simulink model "pendulum_on_a_cart_ctrl"  (R2020a)
settings: Solver=daessc  StartTime=0.0  StopTime=simlength  MaxStep=ts  RelTol=1e-3
values from neighbouring files (symbols this model uses):
  A = [0 1 0 0;      0 -b0*(J1+m1*s1^2)/den  -g*m1^2*s1^2/den b1*m1*s1/den;      0 0 0 1;      0 b0*m1*s1/den g*m1*(m0+m1)*s1/den -b1*(m0+m1)/den]    [init_pendulum_on_a_cart_ctrl.m]
  B = [0 (J1+m1*s1^2)/den 0 -m1*s1/den]'    [init_pendulum_on_a_cart_ctrl.m]
  C = [1 0 0 0; 0 0 1 0]    [init_pendulum_on_a_cart_ctrl.m]
  g = 9.8    [init_pendulum_on_a_cart_ctrl.m]
  Ke = acker(Ae,Be,poles_sf)    [init_pendulum_on_a_cart_ctrl.m]
  L = (place(A',C',poles_obs))'    [init_pendulum_on_a_cart_ctrl.m]
libraries: nesl_utility x6, pendulum_on_a_cart_lib x1
settings Model: Creator=dbagn  LastModifiedBy=dbagn
settings DataIOCC: ReturnWorkspaceOutputs=off

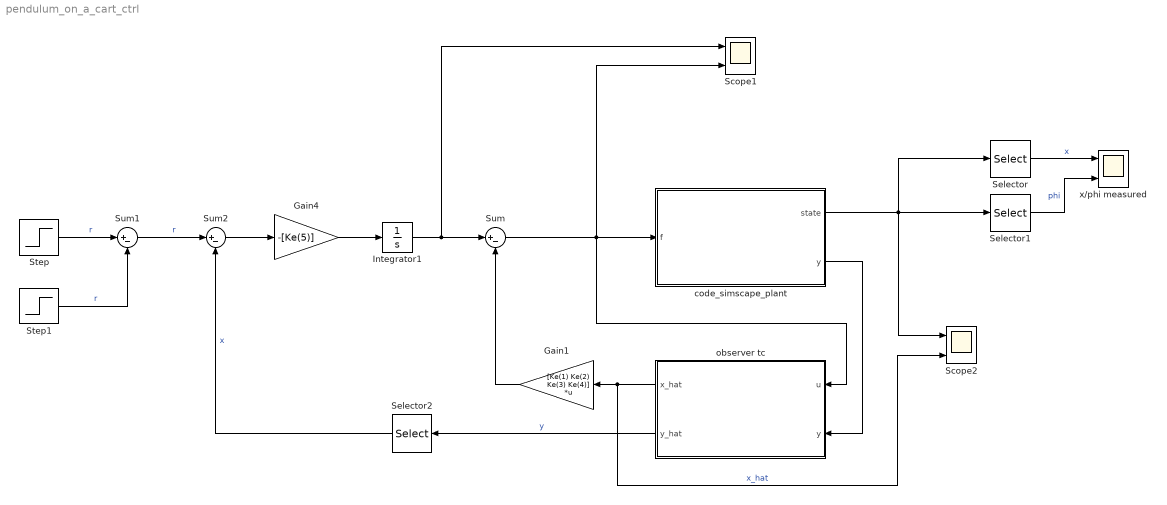
== system pendulum_on_a_cart_ctrl ==
  Gain1 : Gain  Gain=[Ke(1) Ke(2) Ke(3) Ke(4)]  Multiplication=Matrix(K*u)
  Gain4 : Gain  Gain=-[Ke(5)]
  Integrator1 : Integrator
  Scope1 : Scope  NumInputPorts=2
  Scope2 : Scope  NumInputPorts=2
  Selector : Selector  InputPortWidth=4  IndexOptions=Index vector (dialog)  Indices=1  OutputSizes=1
  Selector1 : Selector  InputPortWidth=4  IndexOptions=Index vector (dialog)  Indices=3  OutputSizes=1
  Selector2 : Selector  InputPortWidth=2  IndexOptions=Index vector (dialog)  Indices=1  OutputSizes=1
  Step : Step  SampleTime=0
  Step1 : Step  Time=8  After=2  SampleTime=0
  Sum : Sum  Inputs=|+-
  Sum1 : Sum  Inputs=|+-
  Sum2 : Sum  Inputs=|+-
  "code_simscape_plant " : Subsystem
  observer tc : Subsystem
  x/phi measured : Scope  NumInputPorts=2
  wires:
  Selector/1 -> x/phi measured/1  "x"
  Integrator1/1 -> Sum/1, Scope1/1
  "code_simscape_plant "/2(y) -> observer tc/2(y)
  observer tc/2(y_hat) -> Selector2/1  "y"
  Sum1/1 -> Sum2/1  "r"
  Gain4/1 -> Integrator1/1
  Sum2/1 -> Gain4/1
  Selector1/1 -> x/phi measured/2  "phi"
  Sum/1 -> Scope1/2, observer tc/1(u), "code_simscape_plant "/1(f)
  "code_simscape_plant "/1(state) -> Selector/1, Scope2/1, Selector1/1
  Gain1/1 -> Sum/2
  observer tc/1(x_hat) -> Scope2/2, Gain1/1  "x_hat"
  Selector2/1 -> Sum2/2  "x"
  Step/1 -> Sum1/1  "r"
  Step1/1 -> Sum1/2  "r"

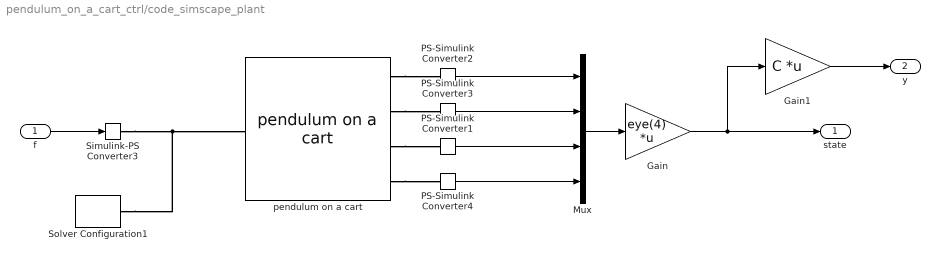
== system pendulum_on_a_cart_ctrl/code_simscape_plant  ==
  f : Inport
  Gain : Gain  Gain=eye(4)  Multiplication=Matrix(K*u)
  Gain1 : Gain  Gain=C  Multiplication=Matrix(K*u)
  Mux : Mux
  PS-Simulink Converter1 : nesl_utility/PS-Simulink Converter  PhysicalDomain=network_engine_domain  SubClassName=ps_output  LeftPortType=input  RightPortType=output  PseudoPeriodic=off  Frequencies=[]  Unit=rad  AffineConversion=on
  PS-Simulink Converter2 : nesl_utility/PS-Simulink Converter  PhysicalDomain=network_engine_domain  SubClassName=ps_output  LeftPortType=input  RightPortType=output  PseudoPeriodic=off  Frequencies=[]  Unit=m  AffineConversion=on
  PS-Simulink Converter3 : nesl_utility/PS-Simulink Converter  PhysicalDomain=network_engine_domain  SubClassName=ps_output  LeftPortType=input  RightPortType=output  PseudoPeriodic=off  Frequencies=[]  Unit=m/s  AffineConversion=on
  PS-Simulink Converter4 : nesl_utility/PS-Simulink Converter  PhysicalDomain=network_engine_domain  SubClassName=ps_output  LeftPortType=input  RightPortType=output  PseudoPeriodic=off  Frequencies=[]  Unit=rad/s  AffineConversion=on
  Simulink-PS Converter3 : nesl_utility/Simulink-PS Converter  PhysicalDomain=network_engine_domain  SubClassName=ps_input  LeftPortType=input  RightPortType=output  PseudoPeriodic=off  Frequencies=[]  NoiseDistribution=none  NoiseParameters=[]  Unit=N  AffineConversion=off  FilteringAndDerivatives=provide  SimscapeFilterOrder=1  InputFilterTimeConstant=0.001  UdotUserProvided=0
  Solver Configuration1 : nesl_utility/Solver Configuration  PhysicalDomain=network_engine_domain  SubClassName=solver  LeftPortType=input  RightPortType=generic  Tones=[]  Harmonics=[]  SimulateNoise=off  Profile=off  UseLocalSampling=off  EnableSwitchedLinearOptims=on  FrequencyDomain=off  UseCCode=off  RelTol=0.001  AbsTol=1e-06  MinStep=1e-09  ToWorkspace=off  RevertToSquareIcSolve=off  NumHomotopyIterations=100  PhasorMode=off  PhasorModeNumHarmonics=1  DoDC=on  ResidualTolerance=1e-09  UseLocalSolver=off  LocalSolverChoice=NE_BACKWARD_EULER_ADVANCER  LocalSolverSampleTime=ts  DoFixedCost=off  MaxNonlinIter=3  MaxModeIter=2  LinearAlgebra=auto  EquationFormulation=NE_TIME_EF  DelaysMemoryBudget=1024  AutomaticFiltering=on  FilteringTimeConstant=0.001  PartitionStorageMethod=AS_NEEDED  PartitionMemoryBudget=1024  PartitionMethod=ROBUST
  pendulum on a cart : pendulum_on_a_cart_lib/pendulum on a cart  m0=m0 kg  m1=m1 kg  J1=J1 kg*m^2  s1=s1 m  b0=b0 N/(m/s)  b1=b1 N*m/(rad/s)  g=g m/s^2  x1_specify=off  x1_priority=High  x1=0 m  x1_nominal_specify=off  x1_nominal_unit=m  x1_nominal_value=1  x2_specify=off  x2_priority=High  x2=0 m/s  x2_nominal_specify=off  x2_nominal_unit=m/s  x2_nominal_value=1  x3_specify=off  x3_priority=High  x3=pi rad  x3_nominal_specify=off  x3_nominal_unit=rad  x3_nominal_value=1  x4_specify=off  x4_priority=High  x4=0 rad/s  x4_nominal_specify=off  x4_nominal_unit=rad/s  x4_nominal_value=1
      settings: InternalSimscapePortConfiguration="{\"Bottom\":[],\"Left\":[{\"id\":\"f\",\"label\":\"f\",\"type\":\"input\"}],\"Right\":[{\"id\":\"x\",\"label\":\"x\",\"type\":\"output\"},{\"id\":\"v\",\"label\":\"v\",\"type\":\"output\"},{\"id\":\"phi\",\"label\":\"phi\",\"type\":\"output\"},{\"id\":\"omega\",\"label\":\"omega\",\"type\":\"output\"}],\"Top\":[]}"
  state : Outport
  y : Outport  Port=2
  wires:
  PS-Simulink Converter2/1 -> Mux/1
  PS-Simulink Converter3/1 -> Mux/2
  f/1 -> Simulink-PS Converter3/1
  PS-Simulink Converter1/1 -> Mux/3
  PS-Simulink Converter4/1 -> Mux/4
  Mux/1 -> Gain/1
  Gain/1 -> Gain1/1, state/1
  Gain1/1 -> y/1
  connections:
  Simulink-PS Converter3/RConn1 -- Solver Configuration1/RConn1 -- pendulum on a cart/LConn1
  pendulum on a cart/RConn1 -- PS-Simulink Converter2/LConn1
  pendulum on a cart/RConn2 -- PS-Simulink Converter3/LConn1
  pendulum on a cart/RConn3 -- PS-Simulink Converter1/LConn1
  pendulum on a cart/RConn4 -- PS-Simulink Converter4/LConn1

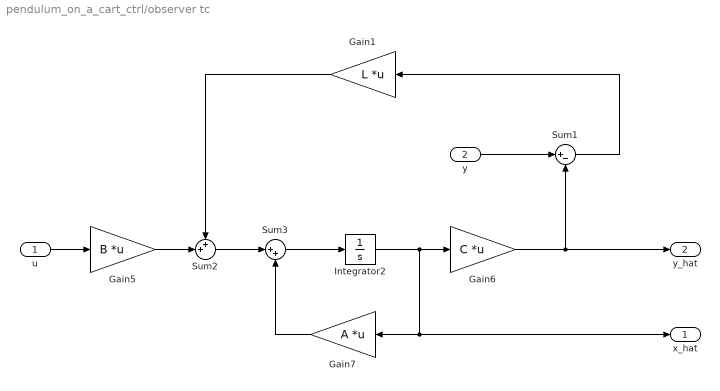
== system pendulum_on_a_cart_ctrl/observer tc ==
  u : Inport
  y : Inport  Port=2
  Gain1 : Gain  Gain=L  Multiplication=Matrix(K*u)
  Gain5 : Gain  Gain=B  Multiplication=Matrix(K*u)
  Gain6 : Gain  Gain=C  Multiplication=Matrix(K*u)
  Gain7 : Gain  Gain=A  Multiplication=Matrix(K*u)
  Integrator2 : Integrator  InitialCondition=[0 0 0 0]
  Sum1 : Sum  Inputs=|+-
  Sum2 : Sum  Inputs=++|
  Sum3 : Sum  Inputs=|++
  x_hat : Outport
  y_hat : Outport  Port=2
  wires:
  Sum2/1 -> Sum3/1
  Integrator2/1 -> x_hat/1, Gain7/1, Gain6/1
  Sum3/1 -> Integrator2/1
  Gain7/1 -> Sum3/2
  y/1 -> Sum1/1
  Gain6/1 -> y_hat/1, Sum1/2
  Sum1/1 -> Gain1/1
  u/1 -> Gain5/1
  Gain1/1 -> Sum2/1
  Gain5/1 -> Sum2/2
